simulink model "hw5_sim"  (R2018b)
settings: Solver=VariableStepAuto  StartTime=0.0  StopTime=5  RelTol=1e-3
values from neighbouring files (symbols this model uses):
  TH = eval(TH)    [hw5_3.m]
undefined symbols (not defined in the file or in its folder): WAM124stateder
settings Model: Creator=arsh  LastModifiedBy=arsh

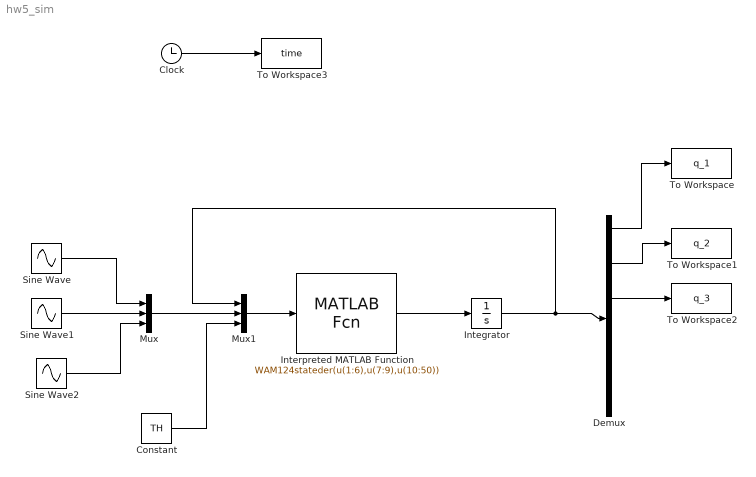
== system hw5_sim ==
  Clock : Clock
  Constant : Constant  Value=TH
  Demux : Demux  Outputs=6
  Integrator : Integrator  InitialCondition=[0; 0; 0; 0; 0; 0]
  Interpreted MATLAB Function : MATLABFcn  MATLABFcn=WAM124stateder(u(1:6),u(7:9),u(10:50))
  Mux : Mux  Inputs=3
  Mux1 : Mux  Inputs=3
  Sine Wave : Sin  SampleTime=0
  Sine Wave1 : Sin  SampleTime=0
  Sine Wave2 : Sin  SampleTime=0
  To Workspace : ToWorkspace  VariableName=q_1  SampleTime=-1
  To Workspace1 : ToWorkspace  VariableName=q_2  SampleTime=-1
  To Workspace2 : ToWorkspace  VariableName=q_3  SampleTime=-1
  To Workspace3 : ToWorkspace  VariableName=time  SampleTime=-1
  wires:
  Sine Wave/1 -> Mux/1
  Sine Wave1/1 -> Mux/2
  Sine Wave2/1 -> Mux/3
  Mux/1 -> Mux1/2
  Constant/1 -> Mux1/3
  Mux1/1 -> Interpreted MATLAB Function/1
  Interpreted MATLAB Function/1 -> Integrator/1
  Integrator/1 -> Demux/1, Mux1/1
  Demux/1 -> To Workspace/1
  Demux/2 -> To Workspace1/1
  Demux/3 -> To Workspace2/1
  Clock/1 -> To Workspace3/1
